simulink model "LineFaultModel1ac"  (R2017b)
settings: Solver=VariableStepAuto  StartTime=0.0  StopTime=0.1  FixedStep=1e-5  MaxStep=1e-4  RelTol=1e-3  EnableMultiTasking=on
undefined symbols (not defined in the file or in its folder): D1, Delta, sps
libraries: powerlib x8, powerlib_meascontrol x6
settings Model: Creator=Rodney  LastModifiedBy=LMS Solution
settings DataIOCC: LimitDataPoints=on  SaveFormat=Array  SignalLoggingSaveFormat=ModelDataLogs
settings OptimizationCC: ExpressionDepthLimit=2147483647  LifeSpan=inf
settings DebuggingCC: UnderspecifiedInitializationDetection=Classic  MergeDetectMultiDrivingBlocksExec=none  SolverPrmCheckMsg=warning  FcnCallInpInsideContextMsg=warning  AllowSymbolicDim=off  StateNameClashWarn=warning  SFUnexpectedBacktrackingDiag=warning  SFNoUnconditionalDefaultTransitionDiag=warning  SFExecutionAtInitializationDiag=none
settings HardwareCC: ProdBitPerPointer=32  ProdBitPerSizeT=32  ProdBitPerPtrDiffT=32  ProdLargestAtomicFloat=None  ProdIntDivRoundTo=Undefined  ProdEndianess=Unspecified  ProdWordSize=32  ProdHWDeviceType=32-bit Generic
settings ModelReferenceCC: PropagateSignalLabelsOutOfModel=off
settings CodeAppCC: StateflowObjectComments=on
settings GRTTargetCC: TargetLangStandard=C89/C90 (ANSI)  GeneratePreprocessorConditionals=Disable all  CombineOutputUpdateFcns=off  GRTInterface=on
settings ConfigComp: CovMetricSettings=dw  CovHtmlReporting=on  CovSaveCumulativeToWorkspaceVar=on  CovSaveSingleToWorkspaceVar=on  CovExternalEMLEnable=off  CovSFcnEnable=off
settings SimscapeCC: SimscapeNormalizeSystem=off

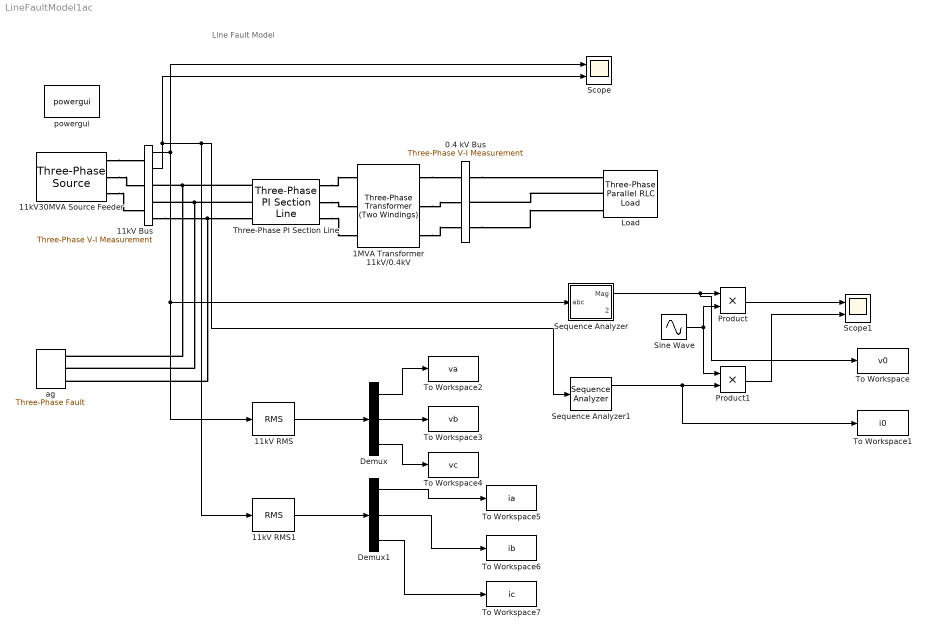
== system LineFaultModel1ac ==
  note: Line Fault Model
  0.4 kV Bus : powerlib/Measurements/Three-Phase V-I Measurement  VoltageMeasurement=no  SetLabelV=off  LabelV=Vabc  Vpu=off  VpuLL=off  CurrentMeasurement=no  SetLabelI=off  LabelI=Iabc  Ipu=off  Pbase=100e6  Vbase=500e3  OutputType=Complex  PhasorSimulation=off  PSBequivalent=0
  11kV Bus : powerlib/Measurements/Three-Phase V-I Measurement  VoltageMeasurement=phase-to-ground  SetLabelV=off  LabelV=Vabc  Vpu=off  VpuLL=off  CurrentMeasurement=yes  SetLabelI=off  LabelI=Iabc  Ipu=off  Pbase=100e6  Vbase=11e3  OutputType=Complex  PhasorSimulation=off  PSBequivalent=0
  11kV RMS : powerlib_meascontrol/Measurements/RMS  TrueRMS=on  Freq=50  RMSInit=4120  Ts=0
  11kV RMS1 : powerlib_meascontrol/Measurements/RMS  TrueRMS=on  Freq=50  RMSInit=5.6  Ts=0
  11kV30MVA Source Feeder : powerlib/Electrical Sources/Three-Phase Source  InternalConnection=Yg  VoltagePhases=off  Voltage=11e3  PhaseAngle=0  Voltage_phases=[25e3 25e3 25e3]/sqrt(3)  PhaseAngles_phases=[0 -120 +120]  Frequency=50  NonIdealSource=on  SpecifyImpedance=on  Resistance=0.8929  Inductance=16.58e-3  ShortCircuitLevel=30e6  BaseVoltage=11e3  XRratio=0.01  BusType=swing  Pref=0  Qref=0  Prefabc=[10e3, 10e3, 10e3]  Qrefabc=[0, 0, 0]  Qmin=-inf  Qmax=inf
  1MVA Transformer 11kV/0.4kV : powerlib/Elements/Three-Phase Transformer (Two Windings)  Winding1Connection=Delta (D1)  Winding2Connection=Yg  CoreType=Three single-phase transformers  SetSaturation=off  Hysteresis=off  DataFile='hysteresis'  SetInitialFlux=off  Measurements=None  UNITS=pu  NominalPower=[ 1e6 , 50 ]  Winding1=[ 11e3 , 0.002 , 0.08 ]  Winding2=[ 0.4e3 , 0.002 , 0.08 ]  Rm=500  Lm=500  L0=0.5  Saturation=[ 0,0 ; 0.0024,1.2 ; 1.0,1.52 ]  InitialFluxes=[ 0.8 , -0.8 , 0.7 ]  MoreParameters=off  BreakLoop=off  DataType=off  TransfoNumber=1
  Demux : Demux  Outputs=3
  Demux1 : Demux  Outputs=3
  Load : powerlib/Elements/Three-Phase Parallel RLC Load  LConnTagsString=A|B|C  Configuration=Y (grounded)  NominalVoltage=1000  Vabc=[1e3 1e3 1e3]  Vabcp=[1e3 1e3 1e3]  NominalFrequency=50  UnbalancedPower=off  ActivePower=10e5  InductivePower=100  CapacitivePower=0  Pabc=[10e3 9e3 11e3]  QLabc=[100 90 110]  QCabc=[100 90 110]  Pabcp=[10e3 9e3 11e3]  QLabcp=[100 90 110]  QCabcp=[100 90 110]  Measurements=None  LoadType=constant Z
  Product : Product
  Product1 : Product
  Scope : Scope  NumInputPorts=2
  Scope1 : Scope  NumInputPorts=2
  Sequence Analyzer : Subsystem  AncestorBlock=powerlib_meascontrol/Measurements/Sequence Analyzer  DialogController=POWERSYS.PowerSysDialog  mask(Sequence Analyzer){Freq=50, n=1, seq=Zero, InInit=[0, 0], Ts=0}
      mask prompts: Freq "Fundamental frequency (Hz):"; n "Harmonic n (1=fundamental):"; seq "Sequence:"; InInit "Initial input [ Mag, Phase (degrees) ]:"; Ts "Sample time:"
      mask help: Compute the positive-, negative-, and zero-sequence components of a three-phase signal.
      mask init:
      | [WantBlockChoice,Ts,sps] = powericon('SequenceAnalyzerInit',gcb,Freq,n,seq,InInit,Ts);
      mask Help: helpview(psbhelp);
      mask TypeOptions seq: Positive | Negative | Zero | Positive Negative Zero
      mask Display:
      | port_label('input',1,'abc')
      | port_label('output',1,'|u|')
      | port_label('output',2,'\angleu', 'texmode', 'on')
  Sequence Analyzer1 : powerlib_meascontrol/Measurements/Sequence Analyzer  Freq=50  n=1  seq=Zero  InInit=[0, 0]  Ts=0
      settings: SourceProductName=Simscape Power Systems  SourceProductBaseCode=PS
  Sine Wave : Sin  Frequency=100*pi  SampleTime=0
  Three-Phase PI Section Line : powerlib/Elements/Three-Phase PI Section Line  LConnTagsString=a|b|c  RConnTagsString=A|B|C  Frequency=50  Resistances=[0.0275 0.275]  Inductances=[0.422/(2*50*pi) 1.169/(2*50*pi)]  Capacitances=[9.483e-9 6.711e-9]  Length=100
      settings: SourceProductName=Simscape Power Systems
  To Workspace : ToWorkspace  VariableName=v0  SampleTime=-1
      settings: MaxDataPoints=1
  To Workspace1 : ToWorkspace  VariableName=i0  SampleTime=-1
      settings: MaxDataPoints=1
  To Workspace2 : ToWorkspace  VariableName=va  SampleTime=-1
      settings: MaxDataPoints=1
  To Workspace3 : ToWorkspace  VariableName=vb  SampleTime=-1
      settings: MaxDataPoints=1
  To Workspace4 : ToWorkspace  VariableName=vc  SampleTime=-1
      settings: MaxDataPoints=1
  To Workspace5 : ToWorkspace  VariableName=ia  SampleTime=-1
      settings: MaxDataPoints=1
  To Workspace6 : ToWorkspace  VariableName=ib  SampleTime=-1
      settings: MaxDataPoints=1
  To Workspace7 : ToWorkspace  VariableName=ic  SampleTime=-1
      settings: MaxDataPoints=1
  ag : powerlib/Elements/Three-Phase Fault  InitialStates=0  FaultA=on  FaultB=off  FaultC=on  GroundFault=off  SwitchTimes=[0.2 0.45]  External=off  SwitchStatus=NaN  FaultResistance=rf  GroundResistance=0.01  SnubberResistance=1e6  SnubberCapacitance=inf  Measurements=Fault voltages
  powergui : powerlib/powergui  Priority=1  SimulationMode=Continuous  SampleTime=50e-6  frequency=60  Iterations=50  frequencyindice=0  Pbase=100e6  ErrMax=1e-4  UnitsV=kV  UnitsW=MW  buscounter=0  FunctionMessages=off  echomessages=off  EnableUseOfTLC=off  CurrentSourceSwitches=on  DisableSnubberDevices=off  DisableRonSwitches=off  DisableVfSwitches=off  DisplayEquations=off  SolverType=Tustin  Interpol=off  ExternalGateDelay=off  methode=off  Ts=0  x0status=blocks  SPID=on  SwTol=0  HookPort=off  RestoreLinks=warning  ResistiveCurrentMeasurement=off  Frange=[0:2:500]  Ylog=off  Xlog=on  ShowGrid=off  save=off  variable=ZData  structure=0  ZoomFFT=off  StartTime=0.0  cycles=1  DisplayStyle=1  fundamental=60  FreqAxis=off  MaxFrequency=1000  frequencyindicesteady=1  RmsSteady=1  display=off
  wires:
  11kV Bus/2 -> 11kV RMS1/1, Sequence Analyzer1/1, Scope/2
  Demux/1 -> To Workspace2/1
  Demux/2 -> To Workspace3/1
  Demux/3 -> To Workspace4/1
  Demux1/1 -> To Workspace5/1
  Demux1/2 -> To Workspace6/1
  Demux1/3 -> To Workspace7/1
  Sequence Analyzer/1(Mag) -> To Workspace/1, Product/1
  Sine Wave/1 -> Product1/1, Product/2
  Product/1 -> Scope1/1
  Sequence Analyzer1/1 -> To Workspace1/1, Product1/2
  Product1/1 -> Scope1/2
  11kV Bus/1 -> Scope/1, 11kV RMS/1, Sequence Analyzer/1(abc)
  11kV RMS1/1 -> Demux1/1
  11kV RMS/1 -> Demux/1
  connections:
  Load/LConn2 -- 0.4 kV Bus/RConn2
  11kV30MVA Source Feeder/RConn2 -- 11kV Bus/LConn2
  11kV30MVA Source Feeder/RConn1 -- 11kV Bus/LConn1
  11kV30MVA Source Feeder/RConn3 -- 11kV Bus/LConn3
  Three-Phase PI Section Line/LConn1 -- ag/LConn1 -- 11kV Bus/RConn1
  11kV Bus/RConn3 -- ag/LConn3 -- Three-Phase PI Section Line/LConn3
  0.4 kV Bus/RConn1 -- Load/LConn1
  0.4 kV Bus/RConn3 -- Load/LConn3
  Three-Phase PI Section Line/RConn1 -- 1MVA Transformer 11kV/0.4kV/LConn1
  Three-Phase PI Section Line/RConn2 -- 1MVA Transformer 11kV/0.4kV/LConn2
  Three-Phase PI Section Line/RConn3 -- 1MVA Transformer 11kV/0.4kV/LConn3
  1MVA Transformer 11kV/0.4kV/RConn1 -- 0.4 kV Bus/LConn1
  1MVA Transformer 11kV/0.4kV/RConn2 -- 0.4 kV Bus/LConn2
  1MVA Transformer 11kV/0.4kV/RConn3 -- 0.4 kV Bus/LConn3
  Three-Phase PI Section Line/LConn2 -- ag/LConn2 -- 11kV Bus/RConn2

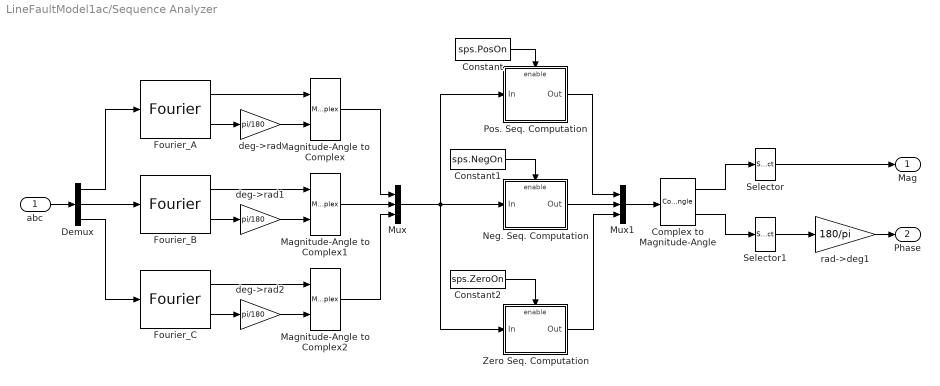
== system LineFaultModel1ac/Sequence Analyzer ==
  abc : Inport  PortDimensions=3  SampleTime=Ts
  Complex to Magnitude-Angle : ComplexToMagnitudeAngle
  Constant : Constant  Value=sps.PosOn
  Constant1 : Constant  Value=sps.NegOn
  Constant2 : Constant  Value=sps.ZeroOn
  Demux : Demux  Outputs=3
  Fourier_A : powerlib_meascontrol/Measurements/Fourier  Freq=sps.Freq  n=sps.n  InInit=sps.Par_Init  Ts=Ts
      settings: SourceProductName=Simscape Power Systems
  Fourier_B : powerlib_meascontrol/Measurements/Fourier  Freq=sps.Freq  n=sps.n  InInit="[sps.Par_Init(1)  sps.Par_Init(2)-120 ]"  Ts=Ts
      settings: SourceProductName=Simscape Power Systems
  Fourier_C : powerlib_meascontrol/Measurements/Fourier  Freq=sps.Freq  n=sps.n  InInit="[sps.Par_Init(1)  sps.Par_Init(2)+120 ]"  Ts=Ts
      settings: SourceProductName=Simscape Power Systems
  Magnitude-Angle to Complex : MagnitudeAngleToComplex
  Magnitude-Angle to Complex1 : MagnitudeAngleToComplex
  Magnitude-Angle to Complex2 : MagnitudeAngleToComplex
  Mux : Mux  Inputs=3
  Mux1 : Mux  Inputs=3
  Neg. Seq. Computation : Subsystem  TreatAsAtomicUnit=on
  Pos. Seq. Computation : Subsystem  TreatAsAtomicUnit=on
  Selector : Selector  InputPortWidth=3  IndexOptions=Index vector (dialog)  Indices=sps.SelectElement  OutputSizes=1
  Selector1 : Selector  InputPortWidth=3  IndexOptions=Index vector (dialog)  Indices=sps.SelectElement  OutputSizes=1
  Zero Seq. Computation : Subsystem  TreatAsAtomicUnit=on
  deg->rad : Gain  Gain=pi/180  SaturateOnIntegerOverflow=on  OutDataTypeStr=Inherit: Same as input  ParamDataTypeStr=Inherit: Same as input
  deg->rad1 : Gain  Gain=pi/180  SaturateOnIntegerOverflow=on  OutDataTypeStr=Inherit: Same as input  ParamDataTypeStr=Inherit: Same as input
  deg->rad2 : Gain  Gain=pi/180  SaturateOnIntegerOverflow=on  OutDataTypeStr=Inherit: Same as input  ParamDataTypeStr=Inherit: Same as input
  rad->deg1 : Gain  Gain=180/pi  SaturateOnIntegerOverflow=on  OutDataTypeStr=Inherit: Same as input  ParamDataTypeStr=Inherit: Same as input
  Mag : Outport  SampleTime=Ts  InitialOutput=0
  Phase : Outport  Port=2  SampleTime=Ts  InitialOutput=0
  wires:
  Selector1/1 -> rad->deg1/1
  Magnitude-Angle to Complex2/1 -> Mux/3
  Magnitude-Angle to Complex1/1 -> Mux/2
  Magnitude-Angle to Complex/1 -> Mux/1
  Fourier_C/2 -> deg->rad2/1
  deg->rad2/1 -> Magnitude-Angle to Complex2/2
  Fourier_C/1 -> Magnitude-Angle to Complex2/1
  Fourier_B/2 -> deg->rad1/1
  deg->rad1/1 -> Magnitude-Angle to Complex1/2
  Fourier_B/1 -> Magnitude-Angle to Complex1/1
  deg->rad/1 -> Magnitude-Angle to Complex/2
  Fourier_A/2 -> deg->rad/1
  Fourier_A/1 -> Magnitude-Angle to Complex/1
  Demux/3 -> Fourier_C/1
  Demux/2 -> Fourier_B/1
  Demux/1 -> Fourier_A/1
  abc/1 -> Demux/1
  Constant1/1 -> Neg. Seq. Computation/Enable
  Complex to Magnitude-Angle/2 -> Selector1/1
  Selector/1 -> Mag/1
  Constant2/1 -> Zero Seq. Computation/Enable
  Constant/1 -> Pos. Seq. Computation/Enable
  Complex to Magnitude-Angle/1 -> Selector/1
  Mux1/1 -> Complex to Magnitude-Angle/1
  Zero Seq. Computation/1(Out) -> Mux1/3
  Neg. Seq. Computation/1(Out) -> Mux1/2
  Pos. Seq. Computation/1(Out) -> Mux1/1
  Mux/1 -> Zero Seq. Computation/1(In), Neg. Seq. Computation/1(In), Pos. Seq. Computation/1(In)
  rad->deg1/1 -> Phase/1

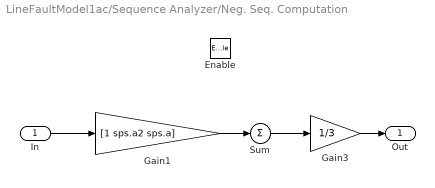
== system LineFaultModel1ac/Sequence Analyzer/Neg. Seq. Computation ==
  In : Inport
  Enable : EnablePort  PropagateVarSize=During execution
  Gain1 : Gain  Gain=[1 sps.a2 sps.a]  SaturateOnIntegerOverflow=on  OutDataTypeStr=Inherit: Same as input  ParamDataTypeStr=Inherit: Same as input
  Gain3 : Gain  Gain=1/3  SaturateOnIntegerOverflow=on  OutDataTypeStr=Inherit: Same as input  ParamDataTypeStr=Inherit: Same as input
  Sum : Sum  Inputs=1  SaturateOnIntegerOverflow=on  InputSameDT=on  OutDataTypeStr=Inherit: Same as first input
  Out : Outport
  wires:
  Gain3/1 -> Out/1
  In/1 -> Gain1/1
  Sum/1 -> Gain3/1
  Gain1/1 -> Sum/1

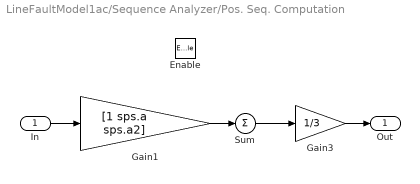
== system LineFaultModel1ac/Sequence Analyzer/Pos. Seq. Computation ==
  In : Inport
  Enable : EnablePort  PropagateVarSize=During execution
  Gain1 : Gain  Gain=[1 sps.a sps.a2]  SaturateOnIntegerOverflow=on  OutDataTypeStr=Inherit: Same as input  ParamDataTypeStr=Inherit: Same as input
  Gain3 : Gain  Gain=1/3  SaturateOnIntegerOverflow=on  OutDataTypeStr=Inherit: Same as input  ParamDataTypeStr=Inherit: Same as input
  Sum : Sum  Inputs=1  SaturateOnIntegerOverflow=on  InputSameDT=on  OutDataTypeStr=Inherit: Same as first input
  Out : Outport
  wires:
  Gain3/1 -> Out/1
  In/1 -> Gain1/1
  Sum/1 -> Gain3/1
  Gain1/1 -> Sum/1

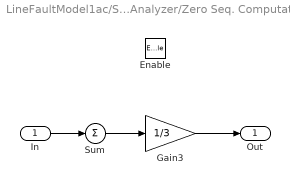
== system LineFaultModel1ac/Sequence Analyzer/Zero Seq. Computation ==
  In : Inport
  Enable : EnablePort  PropagateVarSize=During execution
  Gain3 : Gain  Gain=1/3  SaturateOnIntegerOverflow=on  OutDataTypeStr=Inherit: Same as input  ParamDataTypeStr=Inherit: Same as input
  Sum : Sum  Inputs=1  SaturateOnIntegerOverflow=on  InputSameDT=on  OutDataTypeStr=Inherit: Same as first input
  Out : Outport
  wires:
  Gain3/1 -> Out/1
  In/1 -> Sum/1
  Sum/1 -> Gain3/1
